simulink model "Simulink_model_3Dcube"  (R2024b)
settings: Solver=FixedStepAuto  StartTime=0.0  StopTime=35  FixedStep=0.01  RelTol=1e-3
settings Model: Creator=apple  LastModifiedBy=apple

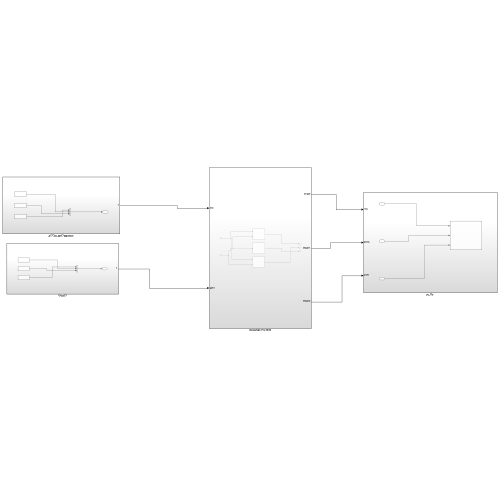
[thumbnail: Simulink's stored preview of the top-level diagram]
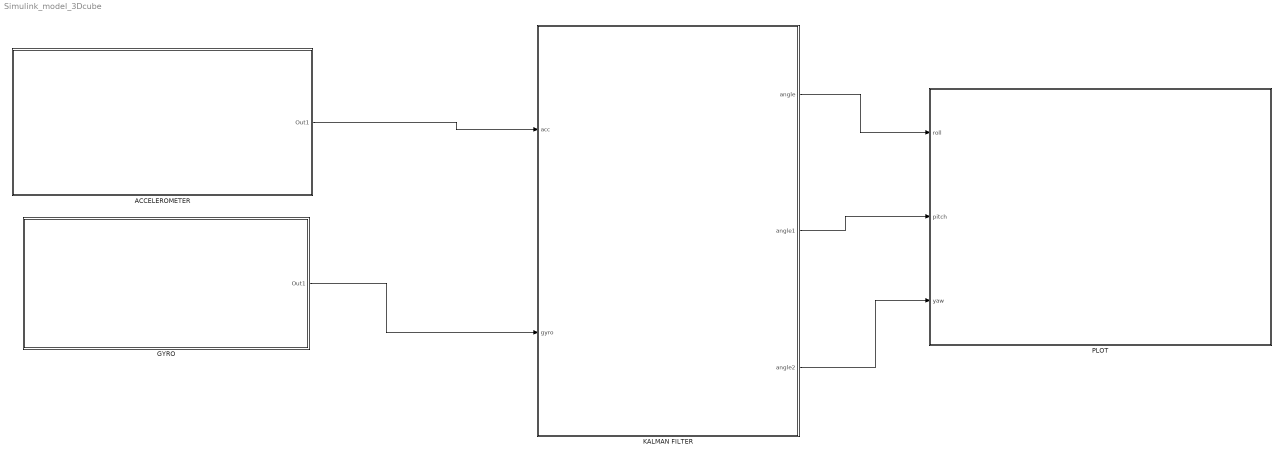
== system Simulink_model_3Dcube ==
  ACCELEROMETER : Subsystem
  GYRO : Subsystem
  KALMAN FILTER : Subsystem
  PLOT : Subsystem
  wires:
  ACCELEROMETER/1(Out1) -> KALMAN FILTER/1(acc)
  GYRO/1(Out1) -> KALMAN FILTER/2(gyro)
  KALMAN FILTER/1(angle) -> PLOT/1(roll)
  KALMAN FILTER/2(angle1) -> PLOT/2(pitch)
  KALMAN FILTER/3(angle2) -> PLOT/3(yaw)

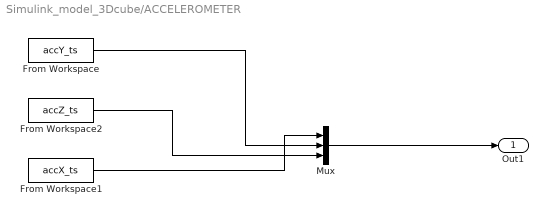
== system Simulink_model_3Dcube/ACCELEROMETER ==
  From Workspace : FromWorkspace  VariableName=accY_ts
  From Workspace1 : FromWorkspace  VariableName=accX_ts
  From Workspace2 : FromWorkspace  VariableName=accZ_ts
  Mux : Mux  Inputs=3
  Out1 : Outport
  wires:
  Mux/1 -> Out1/1
  From Workspace1/1 -> Mux/1
  From Workspace2/1 -> Mux/3
  From Workspace/1 -> Mux/2

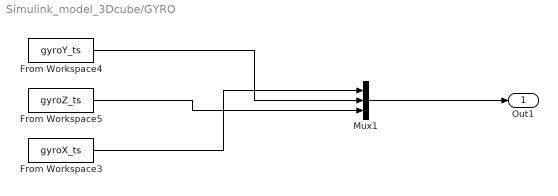
== system Simulink_model_3Dcube/GYRO ==
  From Workspace3 : FromWorkspace  VariableName=gyroX_ts
  From Workspace4 : FromWorkspace  VariableName=gyroY_ts
  From Workspace5 : FromWorkspace  VariableName=gyroZ_ts
  Mux1 : Mux  Inputs=3
  Out1 : Outport
  wires:
  From Workspace4/1 -> Mux1/2
  From Workspace3/1 -> Mux1/1
  Mux1/1 -> Out1/1
  From Workspace5/1 -> Mux1/3

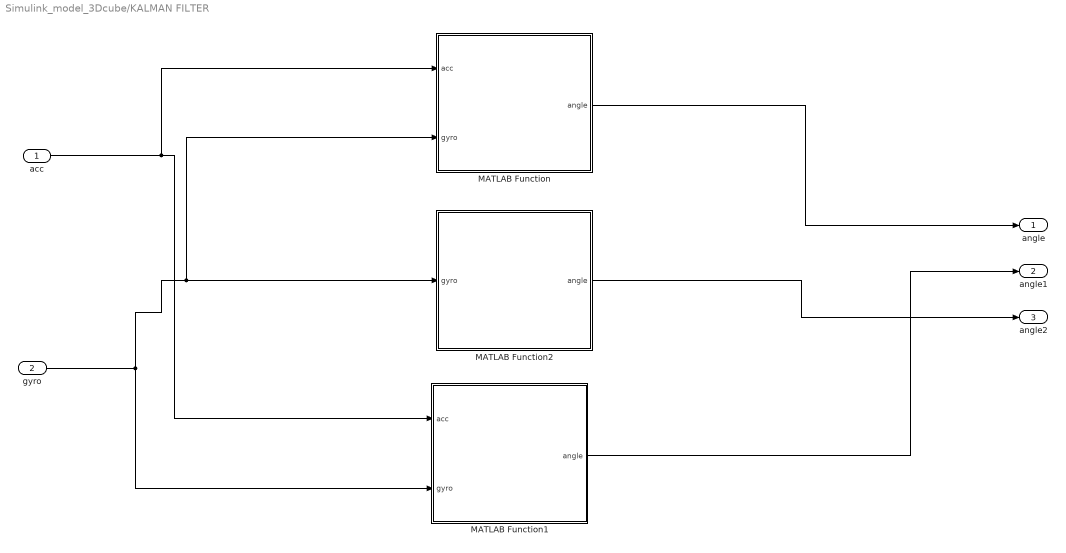
== system Simulink_model_3Dcube/KALMAN FILTER ==
  acc : Inport
  gyro : Inport  Port=2
  MATLAB Function : MATLAB Function  TreatAsAtomicUnit=on
  MATLAB Function1 : MATLAB Function  TreatAsAtomicUnit=on
  MATLAB Function2 : MATLAB Function  TreatAsAtomicUnit=on
  angle : Outport
  angle1 : Outport  Port=2
  angle2 : Outport  Port=3
  wires:
  MATLAB Function/1(angle) -> angle/1
  MATLAB Function2/1(angle) -> angle2/1
  acc/1 -> MATLAB Function1/1(acc), MATLAB Function/1(acc)
  MATLAB Function1/1(angle) -> angle1/1
  gyro/1 -> MATLAB Function1/2(gyro), MATLAB Function2/1(gyro), MATLAB Function/2(gyro)

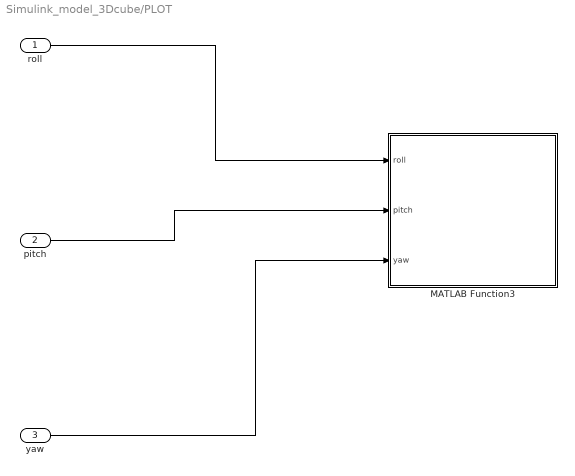
== system Simulink_model_3Dcube/PLOT ==
  roll : Inport
  pitch : Inport  Port=2
  yaw : Inport  Port=3
  MATLAB Function3 : MATLAB Function  TreatAsAtomicUnit=on
  wires:
  yaw/1 -> MATLAB Function3/3(yaw)
  pitch/1 -> MATLAB Function3/2(pitch)
  roll/1 -> MATLAB Function3/1(roll)

== matlab function Simulink_model_3Dcube/KALMAN FILTER/MATLAB Function1 ==
  data: acc input; angle output; gyro input
function angle = kalman_pitch(acc, gyro)
persistent P angle_est
Q = 0.01; R = 0.1; dt = 0.01;
if isempty(P), P = 1; angle_est = 0; end

acc_angle = atan2(-acc(1), sqrt(acc(2)^2 + acc(3)^2));
angle_est = angle_est + gyro(2) * dt;
P = P + Q;

K = P / (P + R);
angle_est = angle_est + K * (acc_angle - angle_est);
P = (1 - K) * P;

angle = angle_est;

== matlab function Simulink_model_3Dcube/KALMAN FILTER/MATLAB Function ==
  data: acc input; angle output; gyro input
function angle = kalman_roll(acc, gyro)
persistent P angle_est
Q = 0.01; R = 0.1; dt = 0.01;
if isempty(P), P = 1; angle_est = 0; end

acc_angle = atan2(acc(2), acc(3));         % roll from acc
angle_est = angle_est + gyro(1) * dt;      % integrate gyro x
P = P + Q;

K = P / (P + R);                            % Kalman gain
angle_est = angle_est + K * (acc_angle - angle_est);
P = (1 - K) * P;

angle = angle_est;

== matlab function Simulink_model_3Dcube/KALMAN FILTER/MATLAB Function2 ==
  data: angle output; gyro input
function angle = kalman_yaw(gyro)
persistent angle_est
dt = 0.01;
if isempty(angle_est), angle_est = 0; end

angle_est = angle_est + gyro(3) * dt;
angle = angle_est;

== matlab function Simulink_model_3Dcube/PLOT/MATLAB Function3 ==
  data: roll input; pitch input; yaw input
function draw(roll, pitch, yaw)
persistent h
if isempty(h)
    h = figure('Name', '3D Cube'); axis equal; grid on;
    xlabel('X'); ylabel('Y'); zlabel('Z'); view(3);
end
clf(h); hold on

Rx = [1 0 0; 0 cos(roll) -sin(roll); 0 sin(roll) cos(roll)];
Ry = [cos(pitch) 0 sin(pitch); 0 1 0; -sin(pitch) 0 cos(pitch)];
Rz = [cos(yaw) -sin(yaw) 0; sin(yaw) cos(yaw) 0; 0 0 1];

R = Rz * Ry * Rx;

verts = [-1 -1 -1; 1 -1 -1; 1 1 -1; -1 1 -1;
         -1 -1  1; 1 -1  1; 1  1  1; -1  1  1]*0.5;
verts = (R * verts')';

faces = [1 2 3 4; 5 6 7 8; 1 5 8 4;
         2 6 7 3; 1 2 6 5; 4 3 7 8];

patch('Vertices', verts, 'Faces', faces, ...
      'FaceColor', [0.6 0.8 1], 'FaceAlpha', 0.6)

quiver3(0,0,0, R(1,1), R(2,1), R(3,1), 1, 'r', 'LineWidth', 2)
quiver3(0,0,0, R(1,2), R(2,2), R(3,2), 1, 'g', 'LineWidth', 2)
quiver3(0,0,0, R(1,3), R(2,3), R(3,3), 1, 'b', 'LineWidth', 2)

xlim([-1 1]); ylim([-1 1]); zlim([-1 1]);
title(sprintf('roll=%.1f deg, pitch=%.1f deg, yaw=%.1f deg', ...
              rad2deg(roll), rad2deg(pitch), rad2deg(yaw)))
